simulink model "sim_file"  (Simulink 9.2)
settings: Solver=VariableStepAuto  StartTime=0.0  StopTime=10.0  RelTol=1e-3
values from neighbouring files (symbols this model uses):
  A = 0.914    [KALMAN.m]    (also in main_cntl.m = eval(A_eq); main_sys.m = double(A_lin); main_sys_klm.m = double(A_lin); main_tf_0.m = A)
  B = 0.25    [KALMAN.m]    (also in main_cntl.m = eval(B_eq); main_sys.m = double(B_lin); main_sys_klm.m = double(B_lin); main_tf_1.m = eval(B))
  C = 0.344    [KALMAN.m]    (also in main_sys.m = double( subs( C) ); main_sys_klm.m = double( subs( C) ); main_tf_0.m = [ 0 , 0  , Ks , ds , -Ks , -ds, 0 ]; main_tf_1.m = C_mes)
  D = zeros(7,2)    [main_sys.m]    (also in main_sys_klm.m = zeros(2,2); main_tf_0.m = [ 0 , 0 ]; main_tf_1.m = zeros(1,1); main_tf_10.m = zeros(2,2))
  Rk = 1    [main_sys_klm.m]    (also in main_tf_10.m; main_tf_11.m; main_tf_12.m = diag([ 10e-8 , 2.25e-8]); main_tf_13.m = diag([ 10e-8 , 2.25e-8]))
  sys_sys = ss(A,B,C,D)    [main_sys.m]    (also in main_sys_klm.m; main_tf_10.m; main_tf_11.m; main_tf_12.m = ss(A_sys,B_sys,C_sys_mod,D_sys_mod))
undefined symbols (not defined in the file or in its folder): Continuous, Time
libraries: ctrlSharedLib x1
settings Model: Creator=eshojaei  LastModifiedBy=eshojaei
settings DataIOCC: LimitDataPoints=off  SaveFormat=Dataset  SignalLoggingSaveFormat=Dataset
settings OptimizationCC: LifeSpan=auto
settings DebuggingCC: UnderspecifiedInitializationDetection=Simplified  MergeDetectMultiDrivingBlocksExec=error  FcnCallInpInsideContextMsg=error  StateNameClashWarn=none  SFUnexpectedBacktrackingDiag=error  SFNoUnconditionalDefaultTransitionDiag=error  SFExecutionAtInitializationDiag=warning
settings HardwareCC: ProdBitPerPointer=64  ProdBitPerSizeT=64  ProdBitPerPtrDiffT=64  ProdLargestAtomicFloat=Float  ProdIntDivRoundTo=Zero  ProdEndianess=LittleEndian  ProdWordSize=64  ProdHWDeviceType=Intel->x86-64 (Windows64)
settings ModelReferenceCC: PropagateSignalLabelsOutOfModel=on
settings SFSimCC: SimUseLocalCustomCode=on
settings RTWCC: RTWUseLocalCustomCode=on
settings GRTTargetCC: TargetLangStandard=C99 (ISO)  GeneratePreprocessorConditionals=Use local settings  CombineOutputUpdateFcns=on  GRTInterface=off
settings ConfigComp: CovMetricSettings=dwe  CovHtmlReporting=off  CovSaveCumulativeToWorkspaceVar=off  CovSaveSingleToWorkspaceVar=off  CovExternalEMLEnable=on

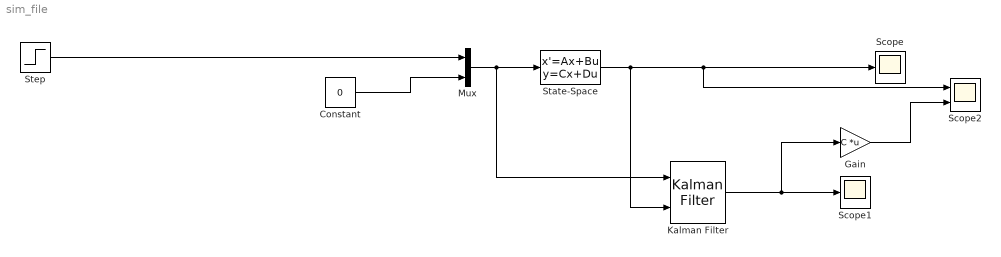
== system sim_file ==
  Constant : Constant  Value=0
  Gain : Gain  Gain=C  Multiplication=Matrix(K*u)
  Kalman Filter : ctrlSharedLib/Kalman Filter  TimeDomain=Continuous-Time  UseCurrentEstimator=off  ModelSource=LTI State-Space Variable  ModelSourceVariable=ss(A,B,C,D)  A=0.95  B=1  C=1  D=0  NumberOfStates=1  NumberOfInputs=1  NumberOfOutputs=1  InitialEstimateSource=Dialog  X0=0  P0=10  UseK=off  UseGH=off  NumberOfProcessNoiseInputs=1  G=1  TimeInvariantG=on  H=0  TimeInvariantH=on  Q=Qk  TimeInvariantQ=on  R=Rk  TimeInvariantR=on  N=0  TimeInvariantN=on  AddInputPort=on  AddEnablePort=off  OutputEstimatedY=off  OutputP=off  Ts=-1
      settings: SourceProductBaseCode=CT
  Mux : Mux  Inputs=2
  Scope : Scope
  Scope1 : Scope
  Scope2 : Scope  NumInputPorts=2
  State-Space : StateSpace  A=sys_sys.A  B=sys_sys.B  C=sys_sys.C  D=sys_sys.D  InitialCondition=0
  Step : Step  Time=.1  After=5  SampleTime=0
  wires:
  Mux/1 -> Kalman Filter/1, State-Space/1
  Constant/1 -> Mux/2
  State-Space/1 -> Kalman Filter/2, Scope2/1, Scope/1
  Kalman Filter/1 -> Gain/1, Scope1/1
  Step/1 -> Mux/1
  Gain/1 -> Scope2/2
